simulink model "AssegnamentoAutovalori"  (R2025b)
settings: Solver=VariableStepAuto  StartTime=0.0  StopTime=10.0  RelTol=1e-3
undefined symbols (not defined in the file): A, B, K_eig, N, n, x_0, x_ref
settings Model: Creator=salvo  LastModifiedBy=salvo

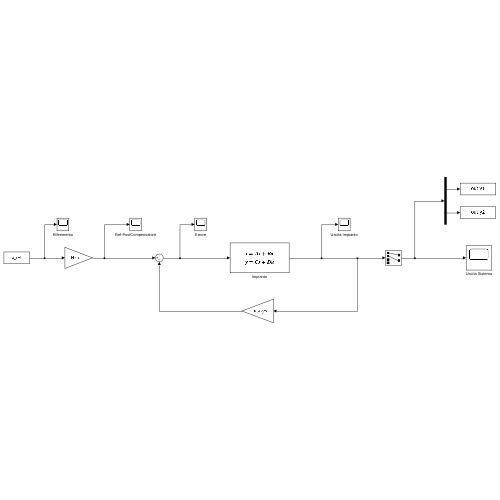
[thumbnail: Simulink's stored preview of the top-level diagram]
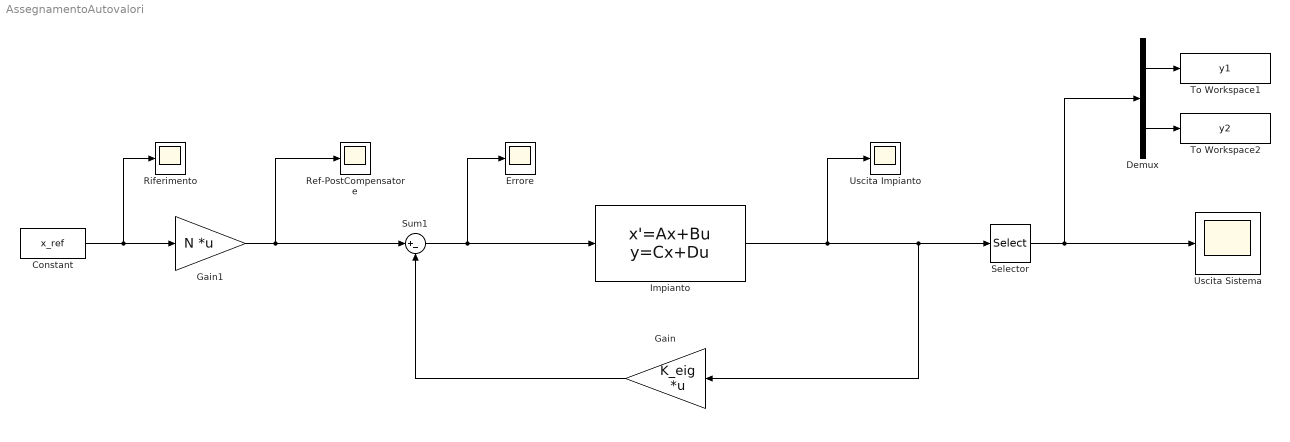
== system AssegnamentoAutovalori ==
  Constant : Constant  Value=x_ref
  Demux : Demux  Outputs=2
  Errore : Scope
      settings: ActiveDisplayYMinimum=-9.7823857380274646  ActiveDisplayYMaximum=52.35097346625993  DataLoggingVariableName=ScopeData2
  Gain : Gain  Gain=K_eig  Multiplication=Matrix(K*u)
  Gain1 : Gain  Gain=N  Multiplication=Matrix(K*u)
  Impianto : StateSpace  A=A  B=B  C=eye(n)  D=zeros(4,2)  InitialCondition=x_0
  Ref-PostCompensatore : Scope
      settings: ActiveDisplayYMinimum=26.450189015066769  ActiveDisplayYMaximum=58.357068541365479  DataLoggingVariableName=ScopeData3
  Riferimento : Scope
      settings: ActiveDisplayYMinimum=0.4375  ActiveDisplayYMaximum=1.0625
  Selector : Selector  InputPortWidth=4  IndexOptions=Index vector (dialog)  Indices=[1 2]  OutputSizes=1
  Sum1 : Sum  Inputs=|+-
  To Workspace1 : ToWorkspace  VariableName=y1  SaveFormat=Timeseries  SampleTime=-1
  To Workspace2 : ToWorkspace  VariableName=y2  SaveFormat=Timeseries  SampleTime=-1
  Uscita Impianto : Scope
      settings: ActiveDisplayYMinimum=-0.1957269181831007  ActiveDisplayYMaximum=0.1578540927139517  DataLoggingVariableName=ScopeData4
  Uscita Sistema : Scope
      settings: ActiveDisplayYMinimum=-0.0327694818957083  ActiveDisplayYMaximum=0.84869745538130825
  wires:
  Impianto/1 -> Uscita Impianto/1, Gain/1, Selector/1
  Selector/1 -> Demux/1, Uscita Sistema/1
  Constant/1 -> Gain1/1, Riferimento/1
  Sum1/1 -> Errore/1, Impianto/1
  Gain/1 -> Sum1/2
  Demux/2 -> To Workspace2/1
  Demux/1 -> To Workspace1/1
  Gain1/1 -> Sum1/1, Ref-PostCompensatore/1
